simulink model "Hypnoz_embedded_continu_v008"  (Simulink 7.7)
settings: Solver=ode3  StartTime=0.0  StopTime=50  FixedStep=Ts  RelTol=1e-3
values from neighbouring files (symbols this model uses):
  A = [-r/L -k/L;km/J -lambda/J]    [SimulationParams.m]
  B = [1/L;0]    [SimulationParams.m]
  Coeff_reprise_obs_I = 1    [SimulationParams.m]
  Coeff_reprise_obs_U = 1    [SimulationParams.m]
  Cs = 196/4    (= 49)    [SimulationParams.m]
  Delt_I2t_max = 1000    [SimulationParams.m]
  Delt_Imot_max = 5    [SimulationParams.m]
  Delt_U2t_max = 1000    [SimulationParams.m]
  Delt_Umot_max = 5    [SimulationParams.m]
  I2t_max = 200000    [SimulationParams.m]
  Imot_max = 220    [SimulationParams.m]
  Isc_max = 300    [SimulationParams.m]
  k = 1/52    (= 0.0192307692308)    [SimulationParams.m]
  Ka = place(Aa,Ba,[p1 p2 p3])    [SimulationParams.m]
  km = 0.16    [SimulationParams.m]
  Koi = K(3:4,:)    [SimulationParams.m]
  Kop = K(1:2,:)    [SimulationParams.m]
  L = 53E-6    (= 5.3e-05)    [SimulationParams.m]
  Masse_vehicule = 850    [SimulationParams.m]
  Pmax_boost = 11750    [SimulationParams.m]
  Pmax_brake = 25000    [SimulationParams.m]
  r = 0.0175    [SimulationParams.m]
  rapport_vitesses = empatement/Rayon_braquage    (= 0.15)    [SimulationParams.m]
  rayon_roue = 0.31    [SimulationParams.m]
  Reduction_electrique = 1/3    (= 0.333333333333)    [SimulationParams.m]
  Th_down = -5    [SimulationParams.m]
  Th_up = 90    [SimulationParams.m]
  to = 0.03    [SimulationParams.m]
  Tr1 = 1000    [SimulationParams.m]
  Tr2 = 1000    [SimulationParams.m]
  Tr6 = 1/Ts    (= 1000)    [SimulationParams.m]
  Ts = 0.001    [SimulationParams.m]
  Ts_sc = 0.005    [SimulationParams.m]
  Umot_max = 96    [SimulationParams.m]
  Usc_max = 192    [SimulationParams.m]
  Usc_min = 96    [SimulationParams.m]
undefined symbols (not defined in the file or in its folder): sigbuilder_block
libraries: simulink x10, simulink_extras x1
(part 2 of 2)

== matlab function SM_System/Electric_propulsion_controler/Control/Control_parameters_monitor1/Erreur_estimation_Tension_g1 ==
  data: Delt_Umot_g input double; Erreur_estimation1 output double; Delt_Umot_d input double; Delt_Umot_max parameter double; Erreur_estimation0 input double; State0 input double; State1 output double; compteur0 input double; Ts_sc parameter double; Delt_U2t_max parameter double; Coeff_reprise_obs_U parameter double; Delt_E0 input double; Tr2 parameter double; Compteur1 output double; Delt_E1 output double
function [Erreur_estimation1,State1,Compteur1, Delt_E1]  = fcn(Delt_Umot_g,Delt_Umot_d, Delt_Umot_max, Erreur_estimation0, State0, compteur0, Ts_sc, Delt_U2t_max,Coeff_reprise_obs_U, Delt_E0, Tr2)

State=State0;
Erreur_estimation=Erreur_estimation0;
Delt_E=Delt_E0;
nc=compteur0;


if(State==0) %fonctionnement normal
    Delt_Umax=max(Delt_Umot_g,Delt_Umot_d);
       if(Delt_Umax > Delt_Umot_max) %si dépassement du Delta_Imot max
           State=1;
       else
        Erreur_estimation=0;
       end
           
elseif(State==1) %erreur detectée
    Delt_Umax=max(Delt_Umot_g,Delt_Umot_d);
    if(Erreur_estimation==0) 
        if(Delt_Umax<Delt_Umot_max && Delt_E>0.3*Delt_U2t_max)%lorsque le Delta_courant retourne en dessous de la valeur seuil, on laisse l'énergie thermique redescendre à 80% de I2t_max avant de retourner dans l'état normal.
            Delt_E=Delt_E-Coeff_reprise_obs_U*(Delt_Umot_max-Delt_Umax)^2*Ts_sc;
        elseif(Delt_Umax<Delt_Umot_max && Delt_E<0.3*Delt_U2t_max)
            Delt_E=0;
            State=0;
        else
            Delt_E=Delt_E+Delt_Umax*Delt_Umax*Ts_sc; %On calcul l'energie emmagasinée dans les cables
        end
        
        if(Delt_E>Delt_U2t_max)
            Erreur_estimation=1;
            nc=0;
        end
        
    elseif(Erreur_estimation==1&&nc>=0) %phase de reprise après erreur
    Delt_Umax=max(Delt_Umot_g,Delt_Umot_d);
        if (Delt_Umax<0.3*Delt_Umot_max)
            nc=nc+1;
            if (nc>=Tr2)
               Erreur_estimation=0;
               State=0;
               Delt_E=0;
               nc=0;
            end
        end
    end
  
else
    State=0;   %%
    Erreur_estimation=0;
    nc=0;
    Delt_E=1;
end

State1=State;
Erreur_estimation1=Erreur_estimation;
Compteur1=nc;
Delt_E1=Delt_E;
end

== matlab function SM_System/Electric_propulsion_controler/Control/Control_parameters_monitor1/Erreur_estimation_courant_g1 ==
  data: Delt_Imot_g input double; Erreur_estimation1 output double; Delt_Imot_d input double; Delt_Imot_max parameter double; Erreur_estimation0 input double; State0 input double; State1 output double; compteur0 input double; Ts_sc parameter double; Delt_I2t_max parameter double; Coeff_reprise_obs_I parameter double; Compteur1 output double; Delt_E0 input double; Delt_E1 output double; Tr1 parameter double
function [Erreur_estimation1,State1,Compteur1, Delt_E1]  = fcn(Delt_Imot_g,Delt_Imot_d, Delt_Imot_max, Erreur_estimation0, State0, compteur0, Ts_sc, Delt_I2t_max,Coeff_reprise_obs_I, Delt_E0, Tr1)

State=State0;
Erreur_estimation=Erreur_estimation0;
Delt_E=Delt_E0;
nc=compteur0;


if(State==0) %fonctionnement normal
    Delt_Imax=max(Delt_Imot_g,Delt_Imot_d);
       if(Delt_Imax > Delt_Imot_max) %si dépassement du Delta_Imot max
           State=1;
       else
        Erreur_estimation=0;
       end
           
elseif(State==1) %erreur detectée
    Delt_Imax=max(Delt_Imot_g,Delt_Imot_d);
    if(Erreur_estimation==0) 
        if(Delt_Imax<Delt_Imot_max && Delt_E>0.3*Delt_I2t_max)%lorsque le Delta_courant retourne en dessous de la valeur seuil, on laisse l'énergie thermique redescendre à 80% de I2t_max avant de retourner dans l'état normal.
            Delt_E=Delt_E-Coeff_reprise_obs_I*(Delt_Imot_max-Delt_Imax)^2*Ts_sc;
        elseif(Delt_Imax<Delt_Imot_max && Delt_E<0.3*Delt_I2t_max)
            Delt_E=0;
            State=0;
        else
            Delt_E=Delt_E+Delt_Imax*Delt_Imax*Ts_sc; %On calcul l'energie emmagasinée dans les cables
        end
        
        if(Delt_E>Delt_I2t_max)
            Erreur_estimation=1;
            nc=0;
        end
        
    elseif(Erreur_estimation==1&&nc>=0) %phase de reprise après erreur
    Delt_Imax=max(Delt_Imot_g,Delt_Imot_d);
        if (Delt_Imax<0.3*Delt_Imot_max)
            nc=nc+1;
            if (nc>=Tr1)
               Erreur_estimation=0;
               State=0;
               Delt_E=0;
               nc=0;
            end
        end
    end
  
else
    State=0;   %%
    Erreur_estimation=0;
    nc=0;
    Delt_E=1;
end

State1=State;
Erreur_estimation1=Erreur_estimation;
Compteur1=nc;
Delt_E1=Delt_E;
end

== matlab function SM_System/Electric_propulsion_controler/Control/Control_general_parameters/erreur_capteur_courant/fcn_precharge ==
  data: enable_capteur_courant output double; enable input double; mode input double; state0 input double; state1 output double
function [enable_capteur_courant, state1]  = fcn(enable, mode,state0)

state=state0;
if(state==0) %fonctionnement normal
    enable_capteur_courant=1;
    if(enable==0)
        state=1;
    end
    
elseif(state==1)
    enable_capteur_courant=0;
    if(mode==0&&enable==1)
        state=0;
    end
else
    state=0;
    enable_capteur_courant=1;
end
state1=state;
end

== matlab function SM_System/Electric_propulsion_controler/Control/Control_parameters_monitor1/Surintensite_g1 ==
  data: Imot input double; Enable_Surint output double; Imot_max parameter double; State0 input double; State1 output double; Enable0 input double; Ts parameter double; I2t_max parameter double; E0 input double; E1 output double
function [Enable_Surint,State1, E1]  = fcn(Imot, Imot_max,State0, Enable0, Ts, I2t_max, E0)

State=State0;
Enable=Enable0;
E=E0;

if(State==0) %fonctionnement normal
      if(Imot > Imot_max) %si dépassement du Imot max
        State=1;
       else
        Enable=1;
        E=0;
       end
           
elseif(State==1) %incrément du compteur
    if(E<I2t_max&&E>=0)
        if(Imot>Imot_max)
            E=E+Imot*Imot*Ts;
        elseif(Imot<0.9*Imot_max)
            E=E-(Imot_max*Imot_max-Imot*Imot)*Ts;
        end
    elseif(E>=I2t_max)
            Enable=0;
            if(Imot<0.9*Imot_max)
            E=E-(Imot_max*Imot_max-Imot*Imot)*Ts;
            end
    else
        State=0;
    end
else
    State=0;   %%
    Enable=1;
    E=0;
end

State1=State;
Enable_Surint=Enable;
E1=E;
end

== matlab function SM_System/Electric_propulsion_controler/Control/Control_parameters_monitor1/Temperature Hacheur_g1 ==
  data: Enable_Th1 output double; Pourcent_Th1 output double; Th_up parameter double; Th_down parameter double; Th1 input double; State0 input double; State1 output double
function [Enable_Th1,Pourcent_Th1,State1]  = fcn(Th_up, Th_down,Th1,State0)

State=State0;
Th=Th1;
Pourcent_Th1=0;

if(State==0) %fonctionnement normal
    Enable_Th1=1;
    Pourcent_Th1=1;
    if((Th>Th_up)) %si la température monte trop
        State=1;
    end
    if((Th<Th_up)&&(Th>Th_down)) % si la température est comprise entre entre Th_up et Th_down, la commande est dégressive
        Pourcent_Th1=(Th_up-Th)/(Th_up-Th_down);
        State=0;
    end
elseif(State==1) % arrêt
    Enable_Th1=0;
    if(Th<=Th_up) % température revenue à un état en dessous de la valeur maximale autorisée
        State=0;
    end
    if((Th<Th_up)&&(Th>Th_down)) % si la température est comprise entre entre Th_up et Ts_down, la commande est dégressive
        Pourcent_Th1=(Th_up-Th)/(Th_up-Th_down);
         Enable_Th1=1;
    end
    if((Th<Th_down)) % si la température est inférieure à Ts_down, on revient à une pleine commande
        Pourcent_Th1=1;
    end
else
    Enable_Th1=0;
    State=0; %%
end
State1=State;
end

== matlab function SM_System/Electric_propulsion_controler/Control/Control_general_parameters/Diff_Capteur_Vitesse ==
  data: Vitesse1 input double; Vitesse2 input double; Erreur_capteur1 output double; Erreur_capteur0 input double; State0 input double; compteur_arret0 input double; State1 output double; Tr6 parameter double; compteur_arret1 output double; mode input double; rapport_vitesses parameter double
function [Erreur_capteur1,State1,compteur_arret1]  = fcn(Vitesse1, Vitesse2, Erreur_capteur0, State0, compteur_arret0, Tr6, mode, rapport_vitesses)

State=State0;
Erreur_capteur=Erreur_capteur0;
nc_arret=compteur_arret0;


if(State==0) %fonctionnement normal
       if(Vitesse1>100&&Vitesse1>Vitesse2)
           if(Vitesse2/Vitesse1<rapport_vitesses)
           State=1;
           else
        Erreur_capteur=1;
        nc_arret=0;
           end
       end
       if(Vitesse2>100&&Vitesse2>Vitesse1)
           if(Vitesse1/Vitesse2<rapport_vitesses)
           State=2;
           else
        Erreur_capteur=1;
        nc_arret=0;
           end
       end
       if(Vitesse1<=0&Vitesse2<=0)
           Erreur_capteur=1;
        nc_arret=0;
       end
       
elseif(State==1) %erreur detectée
    if(Erreur_capteur==1) 
        if(Vitesse2/Vitesse1<rapport_vitesses)% Si la valeur donnée par le capteur ne suit toujours pas la consigne et le temps d'attente n'est pas dépassé
            nc_arret=nc_arret+1; % on incrémente un compteur
           if(nc_arret>Tr6)
                State=10;
           end
         elseif(Vitesse2/Vitesse1>rapport_vitesses)
           if(nc_arret>0)
                nc_arret=nc_arret-1;
           elseif(nc_arret==0)
                State=0;
            end 
        end
    end
    
  
elseif(State==2) %erreur detectée
    if(Erreur_capteur==1) 
        if(Vitesse1/Vitesse2<rapport_vitesses)% Si la valeur donnée par le capteur ne suit toujours pas la consigne et le temps d'attente n'est pas dépassé
            nc_arret=nc_arret+1; % on incrémente un compteur
           if(nc_arret>Tr6)
                State=10;
           end
         elseif(Vitesse1/Vitesse2>rapport_vitesses)
           if(nc_arret>0)
                nc_arret=nc_arret-1;
           elseif(nc_arret==0)
                State=0;
            end 
        end
    end    
    
       
elseif(State==10) % phase de reprise après erreur
     Erreur_capteur=0; % On informe qu'il y a une erreur de capteur
     nc_arret=0;
            if(mode<0.5)
                State=0;
            end
  
else
    State=0;  
    Erreur_capteur=1;
    nc_arret=0;
end

State1=State;
Erreur_capteur1=Erreur_capteur;
compteur_arret1=nc_arret;
end

== matlab function SM_System/Electric_propulsion_controler/Control/Control_general_parameters/fcn_precharge ==
  data: state0 input double; compteur0 input double; state1 output double; enable_start output double; compteur1 output double; mode input double; enable_charge output double; t_prech parameter double
function [state1, enable_start, compteur1, enable_charge] = fcn(state0, compteur0,mode, t_prech)

state=state0;
nc=compteur0;

if(state==0)
enable_start=0;
enable_charge=0;
    if(mode>0.5&&mode<1.5)
        nc=t_prech;
        state=1;
    elseif(mode<0.5)
        state=0;
        nc=0;
    else
        nc=0;
    end
    
elseif(state==1)
enable_start=0;
enable_charge=1;
    if(mode<0.5)
        state=0;
    elseif(nc>0)
        nc=nc-1;
    else
        state=2;
    end
       
elseif(state==2)
    enable_start=1;
    enable_charge=0;
    if((mode<1.5))
        state=0;
    end
else
    enable_start=0;
    enable_charge=0;
    state=0;
    nc=0;
end
state1=state;
compteur1=nc;
end
